simulink subsystem "alt_control"  (R2021a)
settings: Solver=VariableStepAuto  StartTime=0.0  StopTime=10.0  RelTol=1e-3
undefined symbols (not defined in the file or in its folder): C_alt
libraries: simulink x1
settings Model: Creator=EpEp  LastModifiedBy=EpEp

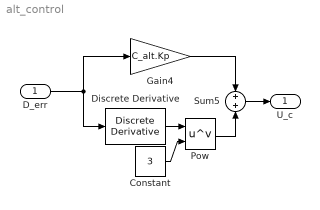
== system alt_control ==
  D_err : Inport
  Constant : Constant  Value=3
  Discrete Derivative : simulink/Quick Insert/Discrete/Discrete Derivative  gainval=-0.08445  ICPrevScaledInput=0.0  OutMin=[]  OutMax=[]  OutDataType=fixdt(1, 16)  OutScaling=2^-10  DoSatur=off
      settings: SourceProductBaseCode=SL
  Gain4 : Gain  Gain=C_alt.Kp
  Pow : Math  Operator=pow  RndMeth=Zero  SaturateOnIntegerOverflow=on
  Sum5 : Sum  Inputs=+|+
  U_c : Outport
  wires:
  D_err/1 -> Discrete Derivative/1, Gain4/1
  Sum5/1 -> U_c/1
  Gain4/1 -> Sum5/1
  Pow/1 -> Sum5/2
  Discrete Derivative/1 -> Pow/1
  Constant/1 -> Pow/2
